simulink model "matlab_model"  (Simulink 8.3)
settings: Solver=ode45  StartTime=0.0  StopTime=10  RelTol=1e-3
InitFcn:
  | sfunction_build
settings Model: Creator=User  LastModifiedBy=mfili
settings OptimizationCC: ExpressionDepthLimit=2147483647
settings DebuggingCC: FcnCallInpInsideContextMsg=UseLocalSettings

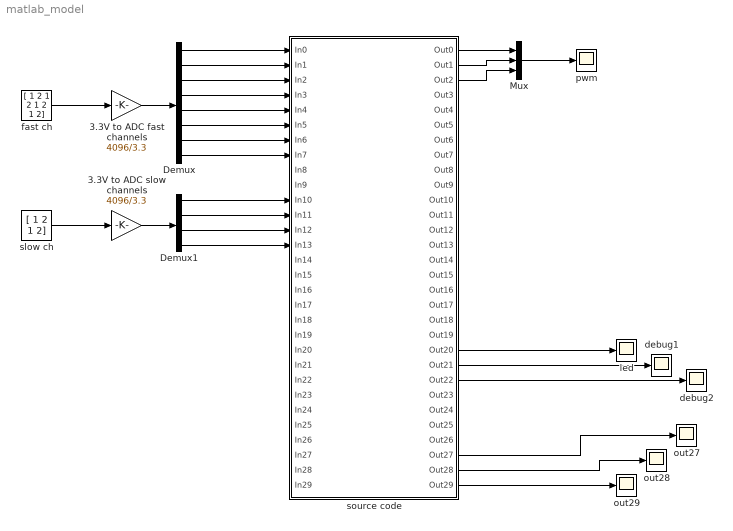
== system matlab_model ==
  3.3V to ADC fast channels : Gain  Gain=4096/3.3
  3.3V to ADC slow channels : Gain  Gain=4096/3.3
  Demux : Demux  Outputs=8
  Demux1 : Demux
  Mux : Mux  Inputs=3
  debug1 : Scope
      settings: SaveName=ScopeData5
  debug2 : Scope
      settings: SaveName=ScopeData6
  fast ch : Constant  Value=[ 1 2 1 2 1 2 1 2]
  led : Scope
      settings: SaveName=ScopeData3
  out27 : Scope
      settings: TimeRange=1  YMin=-0.2  YMax=1.2
  out28 : Scope
      settings: SaveName=ScopeData4
  out29 : Scope
      settings: SaveName=ScopeData2
  pwm : Scope
  slow ch : Constant  Value=[ 1 2 1 2]
  source code : Subsystem
  wires:
  source code/28(Out27) -> out27/1
  source code/29(Out28) -> out28/1
  source code/30(Out29) -> out29/1
  source code/21(Out20) -> led/1
  source code/2(Out1) -> Mux/2
  source code/1(Out0) -> Mux/1
  source code/3(Out2) -> Mux/3
  Mux/1 -> pwm/1
  source code/22(Out21) -> debug1/1
  source code/23(Out22) -> debug2/1
  Demux/1 -> source code/1(In0)
  Demux/2 -> source code/2(In1)
  Demux/3 -> source code/3(In2)
  Demux/4 -> source code/4(In3)
  Demux/5 -> source code/5(In4)
  Demux/6 -> source code/6(In5)
  Demux/7 -> source code/7(In6)
  Demux/8 -> source code/8(In7)
  3.3V to ADC fast channels/1 -> Demux/1
  Demux1/1 -> source code/11(In10)
  Demux1/2 -> source code/12(In11)
  Demux1/3 -> source code/13(In12)
  Demux1/4 -> source code/14(In13)
  3.3V to ADC slow channels/1 -> Demux1/1
  slow ch/1 -> 3.3V to ADC slow channels/1
  fast ch/1 -> 3.3V to ADC fast channels/1

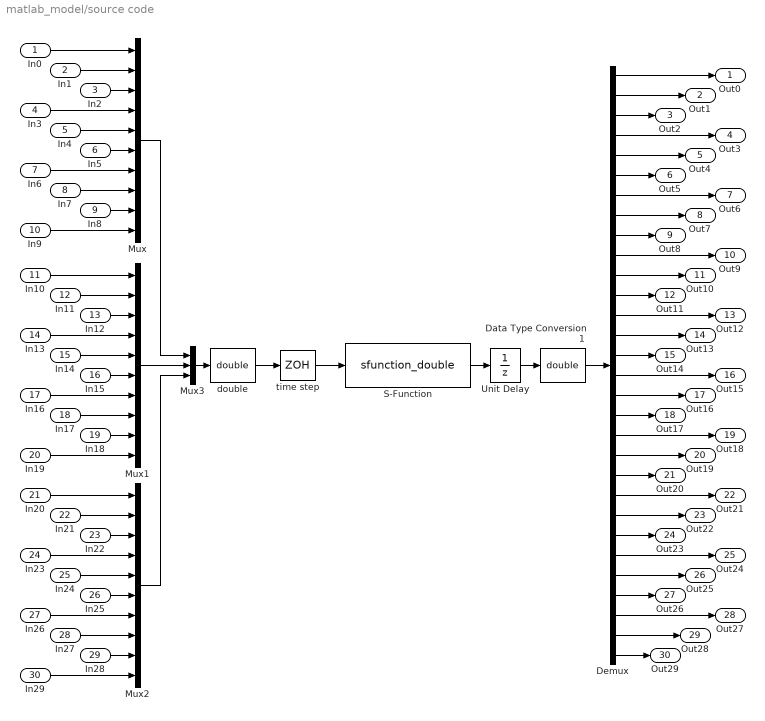
== system matlab_model/source code ==
  In0 : Inport
  In1 : Inport  Port=2
  In2 : Inport  Port=3
  In3 : Inport  Port=4
  In4 : Inport  Port=5
  In5 : Inport  Port=6
  In6 : Inport  Port=7
  In7 : Inport  Port=8
  In8 : Inport  Port=9
  In9 : Inport  Port=10
  In10 : Inport  Port=11
  In11 : Inport  Port=12
  In12 : Inport  Port=13
  In13 : Inport  Port=14
  In14 : Inport  Port=15
  In15 : Inport  Port=16
  In16 : Inport  Port=17
  In17 : Inport  Port=18
  In18 : Inport  Port=19
  In19 : Inport  Port=20
  In20 : Inport  Port=21
  In21 : Inport  Port=22
  In22 : Inport  Port=23
  In23 : Inport  Port=24
  In24 : Inport  Port=25
  In25 : Inport  Port=26
  In26 : Inport  Port=27
  In27 : Inport  Port=28
  In28 : Inport  Port=29
  In29 : Inport  Port=30
  Data Type Conversion1 : DataTypeConversion  OutDataTypeStr=double
  Demux : Demux  Outputs=30
  Mux : Mux  Inputs=10
  Mux1 : Mux  Inputs=10
  Mux2 : Mux  Inputs=10
  Mux3 : Mux  Inputs=3
  S-Function : S-Function  FunctionName=sfunction_double  EnableBusSupport=off
  Unit Delay : UnitDelay  SampleTime=-1
  double : DataTypeConversion  OutDataTypeStr=double
  time step : ZeroOrderHold  SampleTime=1/10000
  Out0 : Outport
  Out1 : Outport  Port=2
  Out2 : Outport  Port=3
  Out3 : Outport  Port=4
  Out4 : Outport  Port=5
  Out5 : Outport  Port=6
  Out6 : Outport  Port=7
  Out7 : Outport  Port=8
  Out8 : Outport  Port=9
  Out9 : Outport  Port=10
  Out10 : Outport  Port=11
  Out11 : Outport  Port=12
  Out12 : Outport  Port=13
  Out13 : Outport  Port=14
  Out14 : Outport  Port=15
  Out15 : Outport  Port=16
  Out16 : Outport  Port=17
  Out17 : Outport  Port=18
  Out18 : Outport  Port=19
  Out19 : Outport  Port=20
  Out20 : Outport  Port=21
  Out21 : Outport  Port=22
  Out22 : Outport  Port=23
  Out23 : Outport  Port=24
  Out24 : Outport  Port=25
  Out25 : Outport  Port=26
  Out26 : Outport  Port=27
  Out27 : Outport  Port=28
  Out28 : Outport  Port=29
  Out29 : Outport  Port=30
  wires:
  double/1 -> time step/1
  In9/1 -> Mux/10
  In8/1 -> Mux/9
  In7/1 -> Mux/8
  In6/1 -> Mux/7
  In5/1 -> Mux/6
  In4/1 -> Mux/5
  In3/1 -> Mux/4
  In2/1 -> Mux/3
  In1/1 -> Mux/2
  In0/1 -> Mux/1
  time step/1 -> S-Function/1
  In19/1 -> Mux1/10
  In18/1 -> Mux1/9
  In17/1 -> Mux1/8
  In16/1 -> Mux1/7
  In15/1 -> Mux1/6
  In14/1 -> Mux1/5
  In13/1 -> Mux1/4
  In12/1 -> Mux1/3
  In11/1 -> Mux1/2
  In10/1 -> Mux1/1
  In29/1 -> Mux2/10
  In28/1 -> Mux2/9
  In27/1 -> Mux2/8
  In26/1 -> Mux2/7
  In25/1 -> Mux2/6
  In24/1 -> Mux2/5
  In23/1 -> Mux2/4
  In22/1 -> Mux2/3
  In21/1 -> Mux2/2
  In20/1 -> Mux2/1
  Mux3/1 -> double/1
  Mux/1 -> Mux3/1
  Mux2/1 -> Mux3/3
  Mux1/1 -> Mux3/2
  Demux/1 -> Out0/1
  Demux/2 -> Out1/1
  Demux/3 -> Out2/1
  Demux/4 -> Out3/1
  Demux/5 -> Out4/1
  Demux/6 -> Out5/1
  Demux/7 -> Out6/1
  Demux/8 -> Out7/1
  Demux/9 -> Out8/1
  Demux/10 -> Out9/1
  Demux/11 -> Out10/1
  Demux/12 -> Out11/1
  Demux/13 -> Out12/1
  Demux/14 -> Out13/1
  Demux/15 -> Out14/1
  Demux/16 -> Out15/1
  Demux/17 -> Out16/1
  Demux/18 -> Out17/1
  Demux/19 -> Out18/1
  Demux/20 -> Out19/1
  Demux/21 -> Out20/1
  Demux/22 -> Out21/1
  Demux/23 -> Out22/1
  Demux/24 -> Out23/1
  Demux/25 -> Out24/1
  Demux/26 -> Out25/1
  Demux/27 -> Out26/1
  Demux/28 -> Out27/1
  Demux/29 -> Out28/1
  Demux/30 -> Out29/1
  S-Function/1 -> Unit Delay/1
  Data Type Conversion1/1 -> Demux/1
  Unit Delay/1 -> Data Type Conversion1/1
